simulink model "Driveline_ctrl_sim"  (R2017b)
settings: Solver=ode45  StartTime=0.0  StopTime=10  MaxStep=0.001  RelTol=1e-3
values from neighbouring files (symbols this model uses):
  A = [-ds/(Jf*r^2) ds/(Jf*r) -cs/(Jf*r); ds/(Jc*r) -ds/Jc cs/Jc; 1/r -1 0]    [Driveline_ctrl_design.m]
  B1 = [B H]    [Driveline_ctrl_design.m]
  C = eye(3)    [Driveline_ctrl_design.m]
  D = zeros(3,2)    [Driveline_ctrl_design.m]
  K = [10.2 325.53 1959.1]    [Driveline_ctrl_design.m]
  kr = 906.9    [Driveline_ctrl_design.m]
  x0 = [120 2 0]'    [Driveline_ctrl_design.m]
settings Model: Creator=jofr  LastModifiedBy=jofr
settings DataIOCC: LimitDataPoints=on  SaveFormat=Array  SignalLoggingSaveFormat=ModelDataLogs
settings OptimizationCC: BlockReduction=off  BooleanDataType=off  LifeSpan=inf
settings DebuggingCC: SaveWithParameterizedLinksMsg=none  UnderspecifiedInitializationDetection=Classic  MergeDetectMultiDrivingBlocksExec=none  SignalResolutionControl=TryResolveAllWithWarning  MultiTaskDSMMsg=warning  MultiTaskCondExecSysMsg=none  SFUnexpectedBacktrackingDiag=warning  SFNoUnconditionalDefaultTransitionDiag=warning  SFExecutionAtInitializationDiag=none
settings HardwareCC: ProdBitPerPointer=32  ProdBitPerSizeT=32  ProdBitPerPtrDiffT=32  ProdLargestAtomicFloat=None  ProdIntDivRoundTo=Undefined  ProdEndianess=Unspecified  ProdWordSize=32  ProdHWDeviceType=32-bit Generic  TargetUnknown=on
settings ModelReferenceCC: PropagateSignalLabelsOutOfModel=off
settings CodeAppCC: StateflowObjectComments=on
settings GRTTargetCC: TargetLangStandard=C89/C90 (ANSI)  GeneratePreprocessorConditionals=Disable all
settings ConfigComp: CovMetricSettings=dw  CovHtmlReporting=on  CovSaveCumulativeToWorkspaceVar=on  CovSaveSingleToWorkspaceVar=on  CovExternalEMLEnable=off

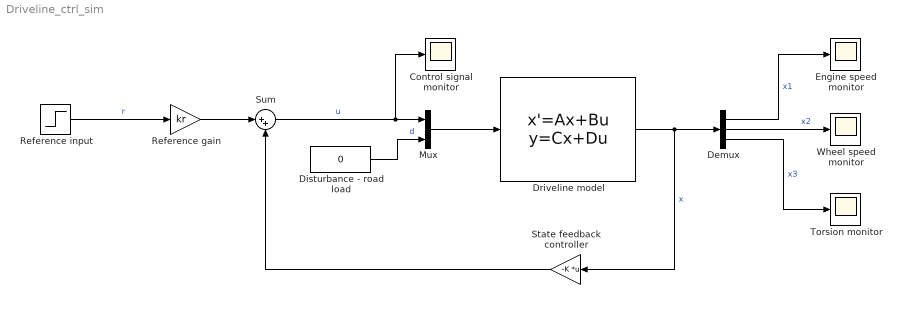
== system Driveline_ctrl_sim ==
  Control signal monitor : Scope
  Demux : Demux  Outputs=3
  Disturbance - road load : Constant  Value=0
  Driveline model : StateSpace  A=A  B=B1  C=C  D=D  InitialCondition=x0
  Engine speed monitor : Scope
  Mux : Mux  Inputs=2
  Reference gain : Gain  Gain=kr
  Reference input : Step  Before=2  After=4  SampleTime=0
  State feedback controller : Gain  Gain=-K  Multiplication=Matrix(K*u)
  Sum : Sum  Inputs=|++
  "Torsion monitor " : Scope
  Wheel speed monitor : Scope
  wires:
  Driveline model/1 -> State feedback controller/1, Demux/1  "x"
  Demux/1 -> Engine speed monitor/1  "x1"
  Demux/2 -> Wheel speed monitor/1  "x2"
  Demux/3 -> "Torsion monitor "/1  "x3"
  Mux/1 -> Driveline model/1
  Disturbance - road load/1 -> Mux/2  "d"
  State feedback controller/1 -> Sum/2
  Reference input/1 -> Reference gain/1  "r"
  Sum/1 -> Control signal monitor/1, Mux/1  "u"
  Reference gain/1 -> Sum/1
